simulink model "Shank_Physics_Model"  (R2024b)
settings: Solver=VariableStepAuto  StartTime=0.0  StopTime=10.0  RelTol=1e-3
undefined symbols (not defined in the file or in its folder): DiscIntNeverNeededParam
settings Model: Creator=shak2  LastModifiedBy=shak2

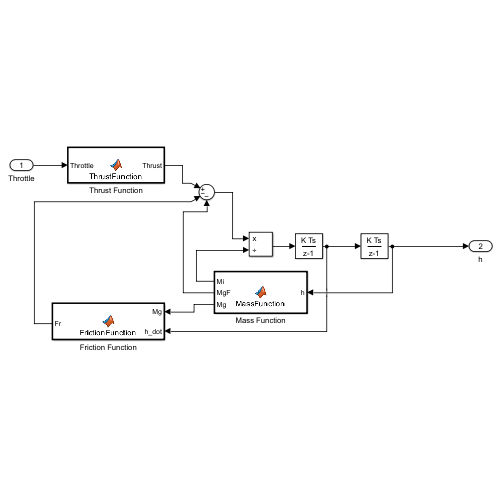
[thumbnail: Simulink's stored preview of the top-level diagram]
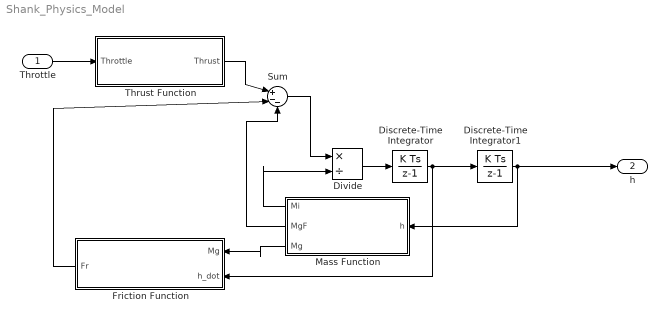
== system Shank_Physics_Model ==
  Throttle : Inport  OutMin=0  OutMax=100  OutDataTypeStr=int8
  Discrete-Time Integrator : DiscreteIntegrator  SampleTime=-1  ICPrevOutput=DiscIntNeverNeededParam  ICPrevScaledInput=DiscIntNeverNeededParam
  Discrete-Time Integrator1 : DiscreteIntegrator  SampleTime=-1  ICPrevOutput=DiscIntNeverNeededParam  ICPrevScaledInput=DiscIntNeverNeededParam
  Divide : Product  Inputs=*/
  Friction Function : MATLAB Function  TreatAsAtomicUnit=on
  Mass Function : MATLAB Function  TreatAsAtomicUnit=on
  Sum : Sum  Inputs=|+--
  Thrust Function : MATLAB Function  TreatAsAtomicUnit=on
  h : Outport  Port=2
  wires:
  Throttle/1 -> Thrust Function/1(Throttle)
  Thrust Function/1(Thrust) -> Sum/1
  Sum/1 -> Divide/1
  Divide/1 -> Discrete-Time Integrator/1
  Discrete-Time Integrator/1 -> Friction Function/2(h_dot), Discrete-Time Integrator1/1
  Discrete-Time Integrator1/1 -> Mass Function/1(h), h/1
  Mass Function/2(MgF) -> Sum/3
  Mass Function/1(Mi) -> Divide/2
  Mass Function/3(Mg) -> Friction Function/1(Mg)
  Friction Function/1(Fr) -> Sum/2

== matlab function Shank_Physics_Model/Thrust Function ==
  data: Throttle input; Thrust output
function Thrust = ThrustFunction(Throttle)

Thrust = Throttle;

== matlab function Shank_Physics_Model/Friction Function ==
  data: Mg input; Fr output; h_dot input
function Fr = FrictionFunction(Mg, h_dot)

Cdf = 0.17; %Coefficient of Dynamic Friction

if h_dot == 0
    Fr = 0.26 * 9.81; %static friction
else
    %% THIS IS A PLACEHOLDER
    N = 0.1 * Mg; %Normal reaction force 
    Fr = (abs(h_dot)/h_dot)*Cdf*N;
end

== matlab function Shank_Physics_Model/Mass Function ==
  data: Mi output; MgF output; h input; Mg output
function [Mi, MgF, Mg] = MassFunction(h)

%Given Masses in Kg
Mm = 0.328; %Motor Mass
Ma = 0.05; %Arm Mass
Mk = 0.15; %Cart Mass

M_constant = Mm + Mk + Ma;

Mc = 0.095*h + 0.532; %mass of cable is function of height

Mg = M_constant + Mc; %gravitational load
Mi = Mg + 0.8 + 0.328; % gravitational + carriage + counterweight + 8 sliders

MgF = Mg * 9.81;
